simulink library "PooliirLib"  (R2022b)
settings: Solver=VariableStepAuto  StartTime=0.0  StopTime=10.0  RelTol=1e-3
undefined symbols (not defined in the file or in its folder): coeffs, maxNumStages, numStages, Row
libraries: PoolIir x4, TuneVar x4, TOP x2, FeaturePath x1, simulink x1
settings Model: Creator=jb10849  LastModifiedBy=jk1043656
settings SolverCC: AlgebraicLoopSolver=TrustRegion
settings DebuggingCC: UnconnectedInputMsg=warning  UnconnectedOutputMsg=warning  UnconnectedLineMsg=warning  SFMachineParentedDataDiag=warning  ArithmeticOperatorsInVariantConditions=warning
settings ModelReferenceCC: EnableRefExpFcnMdlSchedulingChecks=on
settings SFSimCC: SimUseLocalCustomCode=off  CustomCodeUndefinedFunction=UseInterfaceOnly
settings RTWCC: RTWUseLocalCustomCode=off  DLArmComputeVersion=19.05
settings CodeAppCC: StateflowObjectComments=on

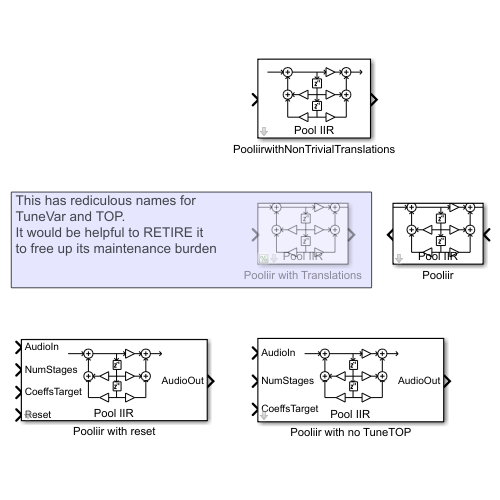
[thumbnail: Simulink's stored preview of the top-level diagram]
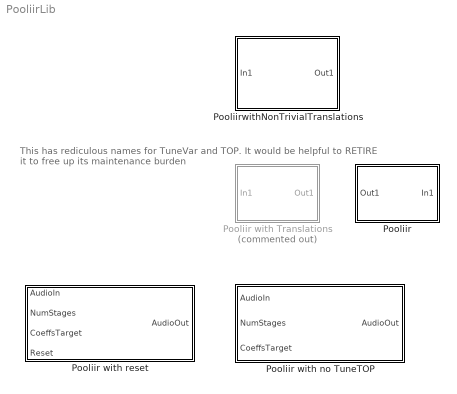
== system PooliirLib ==
  note: This has rediculous names for
      | TuneVar and TOP.
      | It would be helpful to RETIRE it
      | to free up its maintenance burden
  Pooliir : Subsystem  LoadFcn="fprintf(\"\\n ''%s'' block does not support BTC and hence, it will be deprecated soon. Please replace all the active instances of \"\"Pooliir\"\" with an equivalent BTC block.\", gcb);"  mask{maxNumStages=0, numStages=0, coeffs=0, variantType='Generic', FeatureName=filter}
      mask prompts: maxNumStages "Maximum number of stages"; numStages "Number of stages per channel"; coeffs "Coefficient pool"; variantType "Variant"; FeatureName "Filter name/purpose"
      mask init:
      | blkh = gcbh;
      | % Copy discrete mask parameters into a classdef object
      | InnerLinkConfig = PoolIirExternalTranslationConfig;
      | InnerLinkConfig.MaxNumStages = maxNumStages;
      | InnerLinkConfig.DefaultNumStages = numStages;
      | InnerLinkConfig.DefaultSosCoefficients = coeffs;
      | if(isa(variantType, 'char'))
      |     InnerLinkConfig.PoolIir.SelectVariant(variantType);
      | else
      |     error("Please specify the variant in a character format for ''%s''", gcb);
      | end
      mask TypeOptions FeatureName: PoolIirExternalTranslation/FeatureName
      mask Display:
      | [path,w,h] = IconIIR_Mask();
      | 
      | % work in pixels since the icon does not scale
      | pos = get(gcbh,'position');
      | bw = pos(3) - pos(1);
      | bh = pos(4) - pos(2);
      | 
      | % Draw centered icon
      | xAdj = bw/2 - w/2;
      | yAdj = bh/2 - h/2 + 4;
      | for i=1:length(path)
      | %     patch(path(i).x+xAdj, path(i).y+yAdj, path(i).rgb);
      |     plot(path(i).x+xAdj, path(i).y+yAdj);
      | end
      | 
      | % Anchor the corners of the coordinate system
      | patch(0,0,[1 1 1]);
      | patch(bw,bh,[1 1 1]);
      | 
      | % Display some text
      | text(bw/2, bh*0.02,'Pool IIR', ...
      |     'horizontalAlignment','center', ...
      |     'VerticalAlignment','bottom');
  Pooliir with Translations : Subsystem  Commented=on  mask(Bose Pool IIR){maxNumStages=maxNumStages, numStages=numStages, coeffs=single(coeffs), FeatureName=filter}
      mask prompts: maxNumStages "Maximum number of stages"; numStages "Number of stages per channel"; coeffs "Coefficient pool"; FeatureName "Filter name/purpose"
      mask TypeOptions numStages: TOP/Value
      mask TypeOptions coeffs: TOP1/Value
      mask TypeOptions FeatureName: FeaturePath/FeatureName
      mask Display:
      | [path,w,h] = IconIIR_Mask();
      | 
      | % work in pixels since the icon does not scale
      | pos = get(gcbh,'position');
      | bw = pos(3) - pos(1);
      | bh = pos(4) - pos(2);
      | 
      | % Draw centered icon
      | xAdj = bw/2 - w/2;
      | yAdj = bh/2 - h/2 + 4;
      | for i=1:length(path)
      | %     patch(path(i).x+xAdj, path(i).y+yAdj, path(i).rgb);
      |     plot(path(i).x+xAdj, path(i).y+yAdj);
      | end
      | 
      | % Anchor the corners of the coordinate system
      | patch(0,0,[1 1 1]);
      | patch(bw,bh,[1 1 1]);
      | 
      | % Display some text
      | text(bw/2, bh*0.02,'Pool IIR', ...
      |     'horizontalAlignment','center', ...
      |     'VerticalAlignment','bottom');
  Pooliir with no TuneTOP : Subsystem  LoadFcn="fprintf(\"\\n ''%s'' block does not support BTC and hence, it will be deprecated soon. Please replace all the active instances of \"\"Pooliir with no TuneTOP\"\" with an equivalent BTC block.\", gcb);"  mask{maxNumStages=0, alias='Default', variantType='Generic'}
      mask prompts: maxNumStages "Maximum number of stages"; variantType "Variant"
      mask init:
      | blkh = gcbh;
      | % Copy discrete mask parameters into a classdef object
      | InnerLinkConfig = PoolIirConfig;
      | InnerLinkConfig.MaxNumStages = maxNumStages;
      | InnerLinkConfig.Alias = alias;
      | if(isa(variantType, 'char'))
      |     InnerLinkConfig.SelectVariant(variantType);
      | else
      |     error("Please specify the variant in a character format for ''%s''", gcb);
      | end
      mask Display:
      | [path,w,h] = IconIIR_Mask();
      | 
      | % work in pixels since the icon does not scale
      | pos = get(gcbh,'position');
      | bw = pos(3) - pos(1);
      | bh = pos(4) - pos(2);
      | 
      | % Draw centered icon
      | xAdj = bw/2 - w/2;
      | yAdj = bh/2 - h/2 + 4;
      | for i=1:length(path)
      | %     patch(path(i).x+xAdj, path(i).y+yAdj, path(i).rgb);
      |     plot(path(i).x+xAdj, path(i).y+yAdj);
      | end
      | 
      | % Anchor the corners of the coordinate system
      | patch(0,0,[1 1 1]);
      | patch(bw,bh,[1 1 1]);
      | 
      | % Display some text
      | text(bw/2, 1,'Pool IIR', ...
      |     'horizontalAlignment','center', ...
      |     'VerticalAlignment','bottom');
  Pooliir with reset : Subsystem  LoadFcn="fprintf(\"\\n ''%s'' block does not support BTC and hence, it will be deprecated soon. Please replace all the active instances of \"\"Pooliir with reset\"\" with an equivalent BTC block.\", gcb);"  mask{maxNumStages=0, alias=0, variantType='Generic'}
      mask prompts: maxNumStages "Maximum number of stages"; variantType "Variant"
      mask init:
      | InnerLinkConfig = PoolIirConfig;
      | InnerLinkConfig.MaxNumStages = maxNumStages;
      | InnerLinkConfig.Alias = alias;
      | if(isa(variantType, 'char'))
      |     InnerLinkConfig.SelectVariant(variantType);
      | else
      |     error("Please specify the variant in a character format for ''%s''", gcb);
      | end
      mask Display:
      | [path,w,h] = IconIIR_Mask();
      | 
      | % work in pixels since the icon does not scale
      | pos = get(gcbh,'position');
      | bw = pos(3) - pos(1);
      | bh = pos(4) - pos(2);
      | 
      | % Draw centered icon
      | xAdj = bw/2 - w/2;
      | yAdj = bh/2 - h/2 + 4;
      | for i=1:length(path)
      | %     patch(path(i).x+xAdj, path(i).y+yAdj, path(i).rgb);
      |     plot(path(i).x+xAdj, path(i).y+yAdj);
      | end
      | 
      | % Anchor the corners of the coordinate system
      | patch(0,0,[1 1 1]);
      | patch(bw,bh,[1 1 1]);
      | 
      | % Display some text
      | text(bw/2, 1,'Pool IIR', ...
      |     'horizontalAlignment','center', ...
      |     'VerticalAlignment','bottom');
  PooliirwithNonTrivialTranslations : Subsystem  LoadFcn="fprintf(\"\\n ''%s'' block does not support BTC and hence, it will be deprecated soon. Please replace all the active instances of \"\"PooliirwithNonTrivialTranslations\"\" with an equivalent BTC block.\", gcb);"  mask(Bose Pool IIR){maxNumStages=[], numStages=[], sosCoefficients=[], alias='Default', variantType='Generic', FeatureName=filter}
      mask prompts: maxNumStages "Maximum number of stages"; numStages "Number of stages per channel"; sosCoefficients "Coefficient pool"; variantType "Variant"; FeatureName "Filter name/purpose"
      mask init:
      | blkh = gcbh;
      | % Copy discrete mask parameters into a classdef object
      | InnerLinkConfig = PoolIirTunableConfig;
      | InnerLinkConfig.MaxNumStages = maxNumStages;
      | InnerLinkConfig.DefaultNumStages = numStages;
      | InnerLinkConfig.DefaultSosCoefficients = sosCoefficients;
      | InnerLinkConfig.Alias = alias;
      | if(isa(variantType, 'char'))
      |     InnerLinkConfig.SelectVariant(variantType);
      | else
      |     error("Please specify the variant in a character format for ''%s''", gcb);
      | end
      mask TypeOptions FeatureName: InnerLink/FeatureName
      mask Display:
      | [path,w,h] = IconIIR_Mask();
      | 
      | % work in pixels since the icon does not scale
      | pos = get(gcbh,'position');
      | bw = pos(3) - pos(1);
      | bh = pos(4) - pos(2);
      | 
      | % Draw centered icon
      | xAdj = bw/2 - w/2;
      | yAdj = bh/2 - h/2 + 4;
      | for i=1:length(path)
      | %     patch(path(i).x+xAdj, path(i).y+yAdj, path(i).rgb);
      |     plot(path(i).x+xAdj, path(i).y+yAdj);
      | end
      | 
      | % Anchor the corners of the coordinate system
      | patch(0,0,[1 1 1]);
      | patch(bw,bh,[1 1 1]);
      | 
      | % Display some text
      | text(bw/2, 1,'Pool IIR', ...
      |     'horizontalAlignment','center', ...
      |     'VerticalAlignment','bottom');

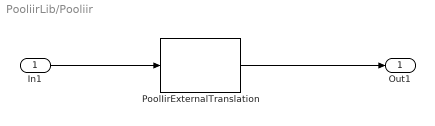
== system PooliirLib/Pooliir ==
  In1 : Inport
  PoolIirExternalTranslation : PoolIir/PoolIirExternalTranslation  Config=InnerLinkConfig  FeatureName=filter
  Out1 : Outport  VectorParamsAs1DForOutWhenUnconnected=off
  wires:
  In1/1 -> PoolIirExternalTranslation/1
  PoolIirExternalTranslation/1 -> Out1/1

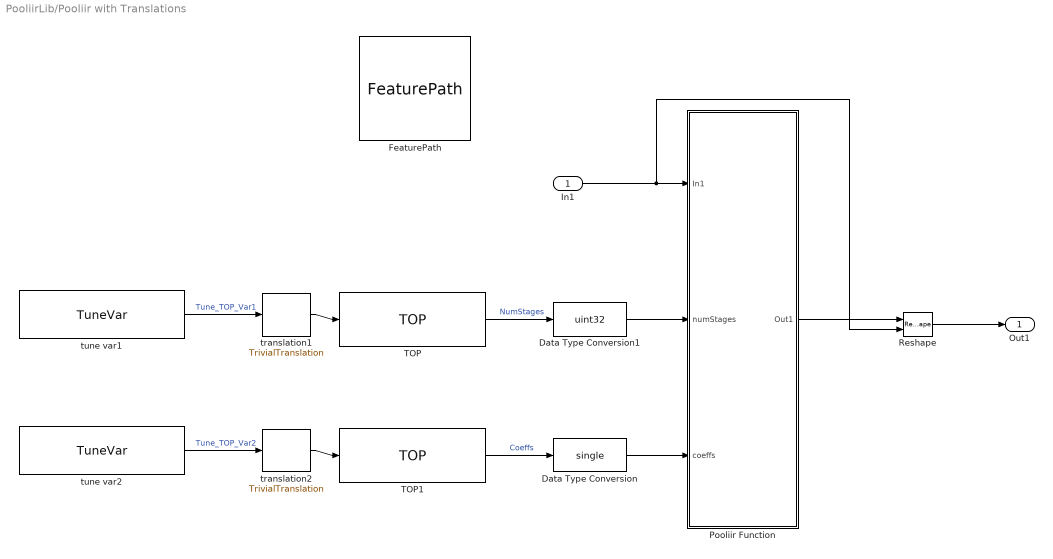
== system PooliirLib/Pooliir with Translations ==
  In1 : Inport
  Data Type Conversion : DataTypeConversion  OutDataTypeStr=single  SaturateOnIntegerOverflow=off  RndMeth=Floor
  Data Type Conversion1 : DataTypeConversion  OutDataTypeStr=uint32  SaturateOnIntegerOverflow=off  RndMeth=Floor
  FeaturePath : FeaturePath/FeaturePath  FeatureName=filter  IsGroup=off  GroupNumber=-1  IsModule=off  TriggerInit=[-205 -51 -90 56]
      settings: SourceProductName=Bose Talaria
  Pooliir Function : Subsystem
  Reshape : Reshape  OutputDimensionality=Derive from reference input port
  TOP : TOP/TOP  TriggerInit=[-225 212 -75 268]  TopName=NumStages  DataTypeOut=single  BankNumber=0  PreOverlay=false  PostOverlay=false  Role=Automatic
      settings: SourceProductName=Bose Talaria
  TOP1 : TOP/TOP  TriggerInit=[-225 352 -75 408]  TopName=Coeffs  DataTypeOut=single  BankNumber=0  PreOverlay=false  PostOverlay=false  Role=Automatic
      settings: SourceProductName=Bose Talaria
  translation1 : TuneVar/TrivialTranslation  TriggerInit=[-305 213 -255 257]
      settings: SourceProductName=Bose Talaria
  translation2 : TuneVar/TrivialTranslation  TriggerInit=[-305 353 -255 397]
      settings: SourceProductName=Bose Talaria
  tune var1 : TuneVar/TuneVar  TuneName=Tune_TOP_Var1  SpecifyMaxSize=off  VariableDim=1 (Row)  MaxSize=[1 1]  TunabilityNumber=1  MinValue=[]  MaxValue=[]  TriggerInit=[-555 210 -385 260]  MaskValue=numStages
      settings: SourceProductName=Bose Talaria
  tune var2 : TuneVar/TuneVar  TuneName=Tune_TOP_Var2  SpecifyMaxSize=off  VariableDim=1 (Row)  MaxSize=[1 1]  TunabilityNumber=1  MinValue=[]  MaxValue=[]  TriggerInit=[-555 350 -385 400]  MaskValue=coeffs
      settings: SourceProductName=Bose Talaria
  Out1 : Outport  VectorParamsAs1DForOutWhenUnconnected=off
  wires:
  Reshape/1 -> Out1/1
  In1/1 -> Pooliir Function/1(In1), Reshape/2
  TOP/1 -> Data Type Conversion1/1  "NumStages"
  TOP1/1 -> Data Type Conversion/1  "Coeffs"
  Pooliir Function/1(Out1) -> Reshape/1
  Data Type Conversion/1 -> Pooliir Function/3(coeffs)
  Data Type Conversion1/1 -> Pooliir Function/2(numStages)
  tune var1/1 -> translation1/1  "Tune_TOP_Var1"
  translation1/1 -> TOP/1
  tune var2/1 -> translation2/1  "Tune_TOP_Var2"
  translation2/1 -> TOP1/1

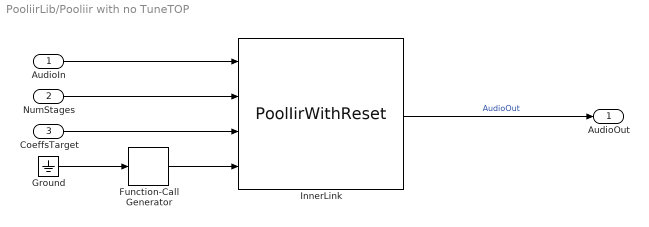
== system PooliirLib/Pooliir with no TuneTOP ==
  AudioIn : Inport
  NumStages : Inport  Port=2
  CoeffsTarget : Inport  Port=3
  Function-Call Generator : simulink/Ports & Subsystems/Function-Call Generator  sample_time=1  numberOfIterations=1  DisallowWideOutput=off  ShowEnablePort=on
  Ground : Ground
  InnerLink : PoolIir/PoolIirWithReset  Config=InnerLinkConfig
  AudioOut : Outport
  wires:
  InnerLink/1 -> AudioOut/1  "AudioOut"
  AudioIn/1 -> InnerLink/1
  NumStages/1 -> InnerLink/2
  CoeffsTarget/1 -> InnerLink/3
  Ground/1 -> Function-Call Generator/1
  Function-Call Generator/1 -> InnerLink/4

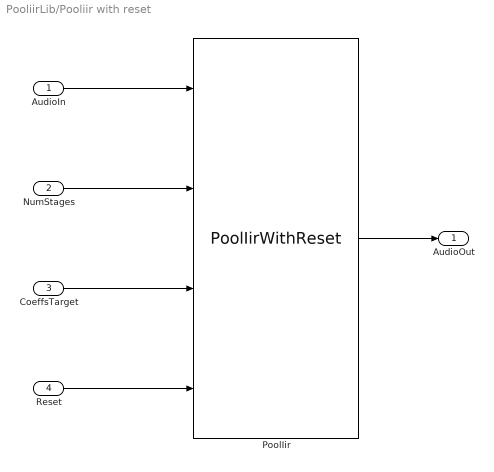
== system PooliirLib/Pooliir with reset ==
  AudioIn : Inport
  NumStages : Inport  Port=2
  CoeffsTarget : Inport  Port=3
  Reset : Inport  Port=4
  PoolIir : PoolIir/PoolIirWithReset  Config=InnerLinkConfig
  AudioOut : Outport  VectorParamsAs1DForOutWhenUnconnected=off
  wires:
  AudioIn/1 -> PoolIir/1
  PoolIir/1 -> AudioOut/1
  NumStages/1 -> PoolIir/2
  CoeffsTarget/1 -> PoolIir/3
  Reset/1 -> PoolIir/4

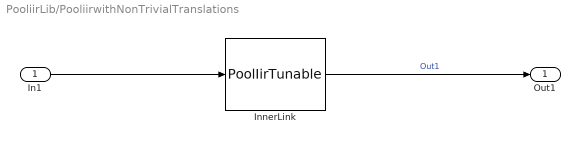
== system PooliirLib/PooliirwithNonTrivialTranslations ==
  In1 : Inport
  InnerLink : PoolIir/PoolIirTunable  FeatureName=filter  Config=InnerLinkConfig
  Out1 : Outport
  wires:
  InnerLink/1 -> Out1/1  "Out1"
  In1/1 -> InnerLink/1

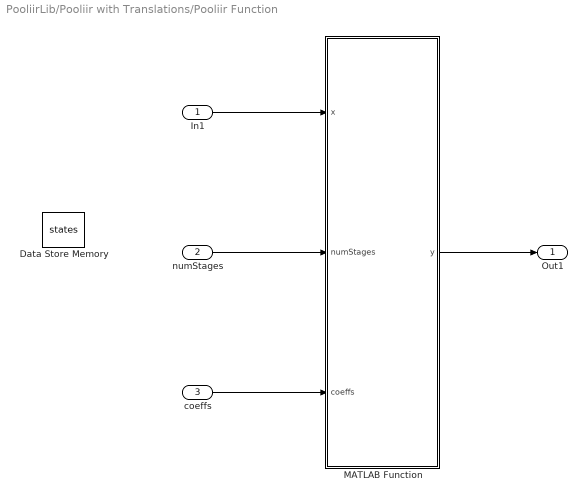
== system PooliirLib/Pooliir with Translations/Pooliir Function ==
  In1 : Inport
  numStages : Inport  Port=2
  coeffs : Inport  Port=3
  Data Store Memory : DataStoreMemory  DataStoreName=states  InitialValue=zeros(1, 2 * maxNumStages)  ShowAdditionalParam=off  OutDataTypeStr=single
  MATLAB Function : MATLAB Function  TreatAsAtomicUnit=on
  Out1 : Outport  VectorParamsAs1DForOutWhenUnconnected=off
  wires:
  MATLAB Function/1(y) -> Out1/1
  numStages/1 -> MATLAB Function/2(numStages)
  In1/1 -> MATLAB Function/1(x)
  coeffs/1 -> MATLAB Function/3(coeffs)

== matlab function PooliirLib/Pooliir with Translations/Pooliir Function/MATLAB Function ==
  data: x input; numStages input uint32; y output single; coeffs input single; states data_store_memory
function y = pooliir_filter(x,numStages, coeffs)
% Extract configuration information from inputs
[frame_size, num_channels] = size(x);

% Initialize variables
global states;

frame_size = uint32(frame_size);
num_channels = uint32(num_channels);

y = pooliir(x, frame_size, num_channels, numStages, coeffs, states);

end

function y = pooliir(x, frameSize, numChannels, numStages, coeffs, states2)
% If code gen'ing, error out if this is not replaced with pooliir.asm
coder.replace('-warnifnoreplacement');

% We have to use a different state buffer than the one passed in.  Matlab
% value objects are passed by value, not by reference, so the saving of
% states here does not work.  The state buffer is still necessary to pass
% allocate in the calling function and pass here in order to trigger CRL.
% This double buffering is annoying, however only happens during
% simulation, not code generation.
% num_states = (length(coeffs) - numChannels) / 2;
% persistent states;
% if isempty(states)
%     states = single(zeros(1, num_states));
% end
global states;
stateIdx = 1;
coeffIdx = 1;

frameMinus1  = frameSize-1;      % number of samples minus one
y     = coder.nullcopy(x); % output matrix

% OUTER LOOP over all channels                 
for cha = 1:numChannels

    % FIRST STAGE
    % prologue: get coefficients, states and input vector 
    % and perform some computations
    
    w1 = states(stateIdx);                          stateIdx = stateIdx+1; 
                        gain = coeffs(coeffIdx);    coeffIdx = coeffIdx+1;
    w2 = states(stateIdx);                          stateIdx = stateIdx-1; 
                        a2   = coeffs(coeffIdx);    coeffIdx = coeffIdx+1;
    xx  = x(1,cha);     a1   = coeffs(coeffIdx);    coeffIdx = coeffIdx+1; 
    xx  = xx*gain;      b2   = coeffs(coeffIdx);    coeffIdx = coeffIdx+1;
    yy  = w1+xx;        b1   = coeffs(coeffIdx);    coeffIdx = coeffIdx+1; 
    w1  = b1*xx;

    % main loop: 5 ops/sample
    for i = 1:frameMinus1
        r  = a1*yy;      w1 = w1+w2;        y(i,cha) = yy;
        q  = b2*xx;      w1 = w1-r;         xx = x(i+1,cha);
        xx = xx*gain;
        w2 = a2*yy;      yy = w1+xx;  
        w1 = b1*xx;      w2 = q-w2; 
    end
    
    % epilogue: drain pipe and write states
    r  = a1*yy;     w1 = w1+w2;             y(frameMinus1+1,cha) = yy;
    q  = b2*xx;     w1 = w1-r; 
    w2 = a2*yy;     states(stateIdx) = w1;  stateIdx = stateIdx+1;
    w2 = q-w2;      states(stateIdx) = w2;  stateIdx = stateIdx+1;              
    % NOTE: asm implementation needs to exit here if it's only
    % one stage, NOTE: all subsequent stages work in-place
      
    for st = 2:numStages(cha)
        % prologue: get coefficients, states and input vector, 
        % and perform some computations
        w1 = states(stateIdx);                      stateIdx = stateIdx+1; 
                            a2 = coeffs(coeffIdx);  coeffIdx = coeffIdx+1;
        w2 = states(stateIdx);                      stateIdx = stateIdx-1; 
                            a1 = coeffs(coeffIdx);  coeffIdx = coeffIdx+1;
        xx = y(1,cha);      b2 = coeffs(coeffIdx);  coeffIdx = coeffIdx+1;
        yy = w1+xx;         b1 = coeffs(coeffIdx);  coeffIdx = coeffIdx+1; 
        w1 = b1*xx;
        
        % main loop: 4 ops/sample
        for i = 1:frameMinus1
            r  = a1*yy;     w1 = w1+w2;         y(i,cha) = yy;
            q  = b2*xx;     w1 = w1-r ;         xx = y(i+1,cha);
            w2 = a2*yy;     yy = w1+xx; 
            w1 = b1*xx;     w2 = q-w2; 
        end
        
        % epilogue: drain pipe and write states
        r  = a1*yy;     w1 = w1+w2;             y(frameMinus1+1,cha) = yy;
        q  = b2*xx;     w1 = w1-r; 
        w2 = a2*yy;     states(stateIdx) = w1;  stateIdx = stateIdx+1;
        w2 = q-w2;      states(stateIdx) = w2;  stateIdx = stateIdx+1;
        
    end
end

end
